simulink library "halin"  (R2021b)
settings: Solver=VariableStepAuto  StartTime=0.0  StopTime=10.0  RelTol=1e-3
undefined symbols (not defined in the file): KHAL_CAN1ABM1E2E_flg, KHAL_CAN1EPB1E2E_flg, KHAL_CAN1EPS1E2E_flg, KHAL_CAN1ESC1E2E_flg, KHAL_CAN1ESC5E2E_flg, KHAL_CAN3BMS1E2E_flg, KHAL_CAN3BMS6E2E_flg, KHAL_CAN3CCU1E2E_flg, KHAL_CAN3CCU2E2E_flg, KHAL_CAN3MCUNF1E2E_flg, KHAL_CAN3MCUNR1E2E_flg, KHAL_CAN3Shifter1E2E_flg, KHAL_CAN3Shifter2E2E_flg, KHAL_CAN6FCM2E2E_flg, KHAL_CAN6FCM4E2E_flg, TRUE
libraries: simulink x645, FVT_lib x212, hcu_lib x59
(part 20 of 23)

== system halin/HAL_IN/CAN3/CCU2/DCDCReady4Pre ==
  DCDCReady4Pre : Inport
  UnitConverter : DataTypeConversion  OutDataTypeStr=uint8
  VHAL_DCDCReady4Pre_flg : Outport
  wires:
  UnitConverter/1 -> VHAL_DCDCReady4Pre_flg/1
  DCDCReady4Pre/1 -> UnitConverter/1

== system halin/HAL_IN/CAN3/CCU2/DCDCTemp ==
  DCDCTemp : Inport
  UnitConverter : DataTypeConversion  OutDataTypeStr=uint8
  convert_in : FVT_lib/hal/convert_in  gain=0.75  offset=-48
  VHAL_DCDCTemp_C : Outport
  wires:
  convert_in/1 -> VHAL_DCDCTemp_C/1
  UnitConverter/1 -> convert_in/1
  DCDCTemp/1 -> UnitConverter/1

== system halin/HAL_IN/CAN3/CCU2/OBCACCurLim ==
  OBC_AC_Cur_Lim : Inport
  UnitConverter : DataTypeConversion  OutDataTypeStr=uint8
  VHAL_OBCACCurLim_enum : Outport
  wires:
  UnitConverter/1 -> VHAL_OBCACCurLim_enum/1
  OBC_AC_Cur_Lim/1 -> UnitConverter/1

== system halin/HAL_IN/CAN3/CCU2/OBCACCurrInf ==
  OBCACCurrInf : Inport
  UnitConverter : DataTypeConversion  OutDataTypeStr=uint16
  convert_in : FVT_lib/hal/convert_in  gain=0.125  offset=-40
  VHAL_OBCACCurrInf_A : Outport
  wires:
  convert_in/1 -> VHAL_OBCACCurrInf_A/1
  UnitConverter/1 -> convert_in/1
  OBCACCurrInf/1 -> UnitConverter/1

== system halin/HAL_IN/CAN3/CCU2/OBCACVoltInf ==
  OBCACVoltInf : Inport
  UnitConverter : DataTypeConversion  OutDataTypeStr=uint16
  convert_in : FVT_lib/hal/convert_in  gain=0.1  offset=0
  VHAL_OBCACVoltInf_V : Outport
  wires:
  convert_in/1 -> VHAL_OBCACVoltInf_V/1
  UnitConverter/1 -> convert_in/1
  OBCACVoltInf/1 -> UnitConverter/1

== system halin/HAL_IN/CAN3/CCU2/OBCEnaSta ==
  OBCEnaSta : Inport
  UnitConverter : DataTypeConversion  OutDataTypeStr=uint8
  VHAL_OBCEnaSta_flg : Outport
  wires:
  UnitConverter/1 -> VHAL_OBCEnaSta_flg/1
  OBCEnaSta/1 -> UnitConverter/1

== system halin/HAL_IN/CAN3/CCU2/OBCFaultSta ==
  OBCFaultSta : Inport
  UnitConverter : DataTypeConversion  OutDataTypeStr=uint8
  VHAL_OBCFaultSta_enum : Outport
  wires:
  UnitConverter/1 -> VHAL_OBCFaultSta_enum/1
  OBCFaultSta/1 -> UnitConverter/1

== system halin/HAL_IN/CAN3/CCU2/OBCPluginSta ==
  OBCPluginSta : Inport
  UnitConverter : DataTypeConversion  OutDataTypeStr=uint8
  VHAL_OBCPluginSta_flg : Outport
  wires:
  UnitConverter/1 -> VHAL_OBCPluginSta_flg/1
  OBCPluginSta/1 -> UnitConverter/1

== system halin/HAL_IN/CAN3/CCU2/OBCReady4Pre ==
  OBCReady4Pre : Inport
  UnitConverter : DataTypeConversion  OutDataTypeStr=uint8
  VHAL_OBCReady4Pre_flg : Outport
  wires:
  UnitConverter/1 -> VHAL_OBCReady4Pre_flg/1
  OBCReady4Pre/1 -> UnitConverter/1

== system halin/HAL_IN/CAN3/CCU2/OBCTemp ==
  OBCTemp : Inport
  UnitConverter : DataTypeConversion  OutDataTypeStr=uint16
  convert_in : FVT_lib/hal/convert_in  gain=0.3  offset=-48
  VHAL_OBCTemp_C : Outport
  wires:
  convert_in/1 -> VHAL_OBCTemp_C/1
  UnitConverter/1 -> convert_in/1
  OBCTemp/1 -> UnitConverter/1

== system halin/HAL_IN/CAN3/CCU2/OBCV2LSta ==
  OBCV2LSta : Inport
  UnitConverter : DataTypeConversion  OutDataTypeStr=uint8
  VHAL_OBCV2LSta_enum : Outport
  wires:
  UnitConverter/1 -> VHAL_OBCV2LSta_enum/1
  OBCV2LSta/1 -> UnitConverter/1

== system halin/HAL_IN/CAN3/CCU2/RCCCU2 ==
  RC_CCU2 : Inport
  UnitConverter : DataTypeConversion  OutDataTypeStr=uint8
  VHAL_RCCCU2_enum : Outport
  wires:
  UnitConverter/1 -> VHAL_RCCCU2_enum/1
  RC_CCU2/1 -> UnitConverter/1

== system halin/HAL_IN/CAN3/EBM1/EBMErrSta ==
  EBMErrSta : Inport
  UnitConverter : DataTypeConversion  OutDataTypeStr=uint8
  VHAL_EBMErrSta_enum : Outport
  wires:
  UnitConverter/1 -> VHAL_EBMErrSta_enum/1
  EBMErrSta/1 -> UnitConverter/1

== system halin/HAL_IN/CAN3/EBM1/EBMRLampSta ==
  EBMRLampSta : Inport
  UnitConverter : DataTypeConversion  OutDataTypeStr=uint8
  VHAL_EBMRLampSta_enum : Outport
  wires:
  UnitConverter/1 -> VHAL_EBMRLampSta_enum/1
  EBMRLampSta/1 -> UnitConverter/1

== system halin/HAL_IN/CAN3/MCU_B_F1/FrActvDmpDisabSta ==
  Fr_ActvDmpDisabSta : Inport
  UnitConverter : DataTypeConversion  OutDataTypeStr=uint8
  VHAL_FrActvDmpDisabSta_flg : Outport
  wires:
  UnitConverter/1 -> VHAL_FrActvDmpDisabSta_flg/1
  Fr_ActvDmpDisabSta/1 -> UnitConverter/1

== system halin/HAL_IN/CAN3/MCU_B_F1/FrEDUDrtSta ==
  Fr_EDUDrtSta : Inport
  UnitConverter : DataTypeConversion  OutDataTypeStr=uint8
  VHAL_FrEDUDrtSta_flg : Outport
  wires:
  UnitConverter/1 -> VHAL_FrEDUDrtSta_flg/1
  Fr_EDUDrtSta/1 -> UnitConverter/1

== system halin/HAL_IN/CAN3/MCU_B_F1/FrEDUOpratingSta ==
  Fr_EDUOpratingSta : Inport
  UnitConverter : DataTypeConversion  OutDataTypeStr=uint8
  VHAL_FrEDUOpratingSta_flg : Outport
  wires:
  UnitConverter/1 -> VHAL_FrEDUOpratingSta_flg/1
  Fr_EDUOpratingSta/1 -> UnitConverter/1

== system halin/HAL_IN/CAN3/MCU_B_F1/FrEDURealTMTq ==
  Fr_EDURealTMTq : Inport
  UnitConverter : DataTypeConversion  OutDataTypeStr=uint16
  convert_in : FVT_lib/hal/convert_in  gain=0.1  offset=-1022
  VHAL_FrEDURealTMTq_Nm : Outport
  wires:
  convert_in/1 -> VHAL_FrEDURealTMTq_Nm/1
  UnitConverter/1 -> convert_in/1
  Fr_EDURealTMTq/1 -> UnitConverter/1

== system halin/HAL_IN/CAN3/MCU_B_F1/FrEDURotateDirction ==
  Fr_EDURotateDirction : Inport
  UnitConverter : DataTypeConversion  OutDataTypeStr=uint8
  VHAL_FrEDURotateDirction_enum : Outport
  wires:
  UnitConverter/1 -> VHAL_FrEDURotateDirction_enum/1
  Fr_EDURotateDirction/1 -> UnitConverter/1

== system halin/HAL_IN/CAN3/MCU_B_F1/FrEDUTqReqFbk ==
  Fr_EDUTqReqFbk : Inport
  UnitConverter : DataTypeConversion  OutDataTypeStr=uint16
  convert_in : FVT_lib/hal/convert_in  gain=1  offset=-1022
  VHAL_FrEDUTqReqFbk_Nm : Outport
  wires:
  convert_in/1 -> VHAL_FrEDUTqReqFbk_Nm/1
  UnitConverter/1 -> convert_in/1
  Fr_EDUTqReqFbk/1 -> UnitConverter/1

== system halin/HAL_IN/CAN3/MCU_B_F1/FrMCUBAT ==
  Fr_MCUBAT : Inport
  UnitConverter : DataTypeConversion  OutDataTypeStr=uint8
  convert_in : FVT_lib/hal/convert_in  gain=0.1  offset=0
  VHAL_FrMCUBAT_V : Outport
  wires:
  convert_in/1 -> VHAL_FrMCUBAT_V/1
  UnitConverter/1 -> convert_in/1
  Fr_MCUBAT/1 -> UnitConverter/1

== system halin/HAL_IN/CAN3/MCU_B_F1/FrMCUDCBusCurr ==
  Fr_MCUDCBusCurr : Inport
  UnitConverter : DataTypeConversion  OutDataTypeStr=uint16
  convert_in : FVT_lib/hal/convert_in  gain=0.1  offset=-1500
  VHAL_FrMCUDCBusCurr_A : Outport
  wires:
  convert_in/1 -> VHAL_FrMCUDCBusCurr_A/1
  UnitConverter/1 -> convert_in/1
  Fr_MCUDCBusCurr/1 -> UnitConverter/1

== system halin/HAL_IN/CAN3/MCU_B_F1/FrMCUDCBusVolt ==
  Fr_MCUDCBusVolt : Inport
  UnitConverter : DataTypeConversion  OutDataTypeStr=uint16
  convert_in : FVT_lib/hal/convert_in  gain=0.1  offset=0
  VHAL_FrMCUDCBusVolt_V : Outport
  wires:
  convert_in/1 -> VHAL_FrMCUDCBusVolt_V/1
  UnitConverter/1 -> convert_in/1
  Fr_MCUDCBusVolt/1 -> UnitConverter/1

== system halin/HAL_IN/CAN3/MCU_B_F1/FrMCUDischrgSta ==
  Fr_MCUDischrgSta : Inport
  UnitConverter : DataTypeConversion  OutDataTypeStr=uint8
  VHAL_FrMCUDischrgSta_flg : Outport
  wires:
  UnitConverter/1 -> VHAL_FrMCUDischrgSta_flg/1
  Fr_MCUDischrgSta/1 -> UnitConverter/1

== system halin/HAL_IN/CAN3/MCU_B_F1/FrMCUEnaSta ==
  Fr_MCUEnaSta : Inport
  UnitConverter : DataTypeConversion  OutDataTypeStr=uint8
  VHAL_FrMCUEnaSta_flg : Outport
  wires:
  UnitConverter/1 -> VHAL_FrMCUEnaSta_flg/1
  Fr_MCUEnaSta/1 -> UnitConverter/1

== system halin/HAL_IN/CAN3/MCU_B_F1/FrMCUErr ==
  Fr_MCUErr : Inport
  UnitConverter : DataTypeConversion  OutDataTypeStr=uint8
  VHAL_FrMCUErr_enum : Outport
  wires:
  UnitConverter/1 -> VHAL_FrMCUErr_enum/1
  Fr_MCUErr/1 -> UnitConverter/1

== system halin/HAL_IN/CAN3/MCU_B_F1/FrMCUIGNsta ==
  Fr_MCUIGN_sta : Inport
  UnitConverter : DataTypeConversion  OutDataTypeStr=uint8
  VHAL_FrMCUIGNsta_flg : Outport
  wires:
  UnitConverter/1 -> VHAL_FrMCUIGNsta_flg/1
  Fr_MCUIGN_sta/1 -> UnitConverter/1

== system halin/HAL_IN/CAN3/MCU_B_F1/FrMCUReady ==
  Fr_MCUReady : Inport
  UnitConverter : DataTypeConversion  OutDataTypeStr=uint8
  VHAL_FrMCUReady_flg : Outport
  wires:
  UnitConverter/1 -> VHAL_FrMCUReady_flg/1
  Fr_MCUReady/1 -> UnitConverter/1

== system halin/HAL_IN/CAN3/MCU_B_F1/FrMCUReady4Pre ==
  Fr_MCUReady4Pre : Inport
  UnitConverter : DataTypeConversion  OutDataTypeStr=uint8
  VHAL_FrMCUReady4Pre_flg : Outport
  wires:
  UnitConverter/1 -> VHAL_FrMCUReady4Pre_flg/1
  Fr_MCUReady4Pre/1 -> UnitConverter/1

== system halin/HAL_IN/CAN3/MCU_B_F1/FrMCUSysSta ==
  Fr_MCUSysSta : Inport
  UnitConverter : DataTypeConversion  OutDataTypeStr=uint8
  VHAL_FrMCUSysSta_enum : Outport
  wires:
  UnitConverter/1 -> VHAL_FrMCUSysSta_enum/1
  Fr_MCUSysSta/1 -> UnitConverter/1

== system halin/HAL_IN/CAN3/MCU_B_F1/FrMCUTemp ==
  Fr_MCUTemp : Inport
  UnitConverter : DataTypeConversion  OutDataTypeStr=uint16
  convert_in : FVT_lib/hal/convert_in  gain=1  offset=-40
  VHAL_FrMCUTemp_C : Outport
  wires:
  convert_in/1 -> VHAL_FrMCUTemp_C/1
  UnitConverter/1 -> convert_in/1
  Fr_MCUTemp/1 -> UnitConverter/1

== system halin/HAL_IN/CAN3/MCU_B_F1/FrMotorAvailTq ==
  Fr_MotorAvailTq : Inport
  UnitConverter : DataTypeConversion  OutDataTypeStr=uint16
  VHAL_FrMotorAvailTq_Nm : Outport
  wires:
  UnitConverter/1 -> VHAL_FrMotorAvailTq_Nm/1
  Fr_MotorAvailTq/1 -> UnitConverter/1

== system halin/HAL_IN/CAN3/MCU_B_F1/FrRegenAvailTq ==
  Fr_RegenAvailTq : Inport
  UnitConverter : DataTypeConversion  OutDataTypeStr=uint16
  convert_in : FVT_lib/hal/convert_in  gain=1  offset=-1022
  VHAL_FrRegenAvailTq_Nm : Outport
  wires:
  convert_in/1 -> VHAL_FrRegenAvailTq_Nm/1
  UnitConverter/1 -> convert_in/1
  Fr_RegenAvailTq/1 -> UnitConverter/1

== system halin/HAL_IN/CAN3/MCU_B_F1/FrTMSpd ==
  Fr_TMSpd : Inport
  UnitConverter : DataTypeConversion  OutDataTypeStr=uint16
  convert_in : FVT_lib/hal/convert_in  gain=1  offset=-18000
  VHAL_FrTMSpd_rpm : Outport
  wires:
  convert_in/1 -> VHAL_FrTMSpd_rpm/1
  UnitConverter/1 -> convert_in/1
  Fr_TMSpd/1 -> UnitConverter/1

== system halin/HAL_IN/CAN3/MCU_B_F1/FrTMTemp ==
  Fr_TMTemp : Inport
  UnitConverter : DataTypeConversion  OutDataTypeStr=uint16
  convert_in : FVT_lib/hal/convert_in  gain=1  offset=-40
  VHAL_FrTMTemp_C : Outport
  wires:
  convert_in/1 -> VHAL_FrTMTemp_C/1
  UnitConverter/1 -> convert_in/1
  Fr_TMTemp/1 -> UnitConverter/1

== system halin/HAL_IN/CAN3/MCU_B_F1/FrTMid ==
  Fr_TMid : Inport
  UnitConverter : DataTypeConversion  OutDataTypeStr=uint16
  convert_in : FVT_lib/hal/convert_in  gain=0.1  offset=-1500
  VHAL_FrTMid_A : Outport
  wires:
  convert_in/1 -> VHAL_FrTMid_A/1
  UnitConverter/1 -> convert_in/1
  Fr_TMid/1 -> UnitConverter/1

== system halin/HAL_IN/CAN3/MCU_B_F1/FrTMiq ==
  Fr_TMiq : Inport
  UnitConverter : DataTypeConversion  OutDataTypeStr=uint16
  convert_in : FVT_lib/hal/convert_in  gain=0.1  offset=-1500
  VHAL_FrTMiq_A : Outport
  wires:
  convert_in/1 -> VHAL_FrTMiq_A/1
  UnitConverter/1 -> convert_in/1
  Fr_TMiq/1 -> UnitConverter/1

== system halin/HAL_IN/CAN3/MCU_B_F1/MCUBFRealPwrKwSta ==
  MCU_B_F_RealPwrKw_Sta : Inport
  UnitConverter : DataTypeConversion  OutDataTypeStr=uint16
  convert_in : FVT_lib/hal/convert_in  gain=0.1  offset=-530
  VHAL_MCUBFRealPwrKwSta_kW : Outport
  wires:
  convert_in/1 -> VHAL_MCUBFRealPwrKwSta_kW/1
  UnitConverter/1 -> convert_in/1
  MCU_B_F_RealPwrKw_Sta/1 -> UnitConverter/1

== system halin/HAL_IN/CAN3/MCU_B_F1/MCUWarnF ==
  MCUWarn_F : Inport
  UnitConverter : DataTypeConversion  OutDataTypeStr=uint8
  VHAL_MCUWarnF_enum : Outport
  wires:
  UnitConverter/1 -> VHAL_MCUWarnF_enum/1
  MCUWarn_F/1 -> UnitConverter/1

== system halin/HAL_IN/CAN3/MCU_B_F2/FrCoolanttempReq ==
  Fr_CoolanttempReq : Inport
  UnitConverter : DataTypeConversion  OutDataTypeStr=uint16
  convert_in : FVT_lib/hal/convert_in  gain=1  offset=-40
  VHAL_FrCoolanttempReq_C : Outport
  wires:
  convert_in/1 -> VHAL_FrCoolanttempReq_C/1
  UnitConverter/1 -> convert_in/1
  Fr_CoolanttempReq/1 -> UnitConverter/1

== system halin/HAL_IN/CAN3/MCU_B_F2/FrFailcode1 ==
  Fr_Failcode1 : Inport
  UnitConverter : DataTypeConversion  OutDataTypeStr=uint8
  VHAL_FrFailcode1_enum : Outport
  wires:
  UnitConverter/1 -> VHAL_FrFailcode1_enum/1
  Fr_Failcode1/1 -> UnitConverter/1

== system halin/HAL_IN/CAN3/MCU_B_F2/FrFailcode2 ==
  Fr_Failcode2 : Inport
  UnitConverter : DataTypeConversion  OutDataTypeStr=uint8
  VHAL_FrFailcode2_enum : Outport
  wires:
  UnitConverter/1 -> VHAL_FrFailcode2_enum/1
  Fr_Failcode2/1 -> UnitConverter/1

== system halin/HAL_IN/CAN3/MCU_B_F2/FrFailcodehistory1 ==
  Fr_Failcodehistory1 : Inport
  UnitConverter : DataTypeConversion  OutDataTypeStr=uint8
  VHAL_FrFailcodehistory1_enum : Outport
  wires:
  UnitConverter/1 -> VHAL_FrFailcodehistory1_enum/1
  Fr_Failcodehistory1/1 -> UnitConverter/1

== system halin/HAL_IN/CAN3/MCU_B_F2/FrFailcodehistory2 ==
  Fr_Failcodehistory2 : Inport
  UnitConverter : DataTypeConversion  OutDataTypeStr=uint8
  VHAL_FrFailcodehistory2_enum : Outport
  wires:
  UnitConverter/1 -> VHAL_FrFailcodehistory2_enum/1
  Fr_Failcodehistory2/1 -> UnitConverter/1

== system halin/HAL_IN/CAN3/MCU_B_F2/FrLLCTemp ==
  Fr_LLCTemp : Inport
  UnitConverter : DataTypeConversion  OutDataTypeStr=uint16
  convert_in : FVT_lib/hal/convert_in  gain=1  offset=-40
  VHAL_FrLLCTemp_C : Outport
  wires:
  convert_in/1 -> VHAL_FrLLCTemp_C/1
  UnitConverter/1 -> convert_in/1
  Fr_LLCTemp/1 -> UnitConverter/1

== system halin/HAL_IN/CAN3/MCU_B_F2/FrLLCflowReq ==
  Fr_LLCflowReq : Inport
  UnitConverter : DataTypeConversion  OutDataTypeStr=uint8
  convert_in : FVT_lib/hal/convert_in  gain=0.25  offset=0
  VHAL_FrLLCflowReq_Lpmin : Outport
  wires:
  convert_in/1 -> VHAL_FrLLCflowReq_Lpmin/1
  UnitConverter/1 -> convert_in/1
  Fr_LLCflowReq/1 -> UnitConverter/1

== system halin/HAL_IN/CAN3/MCU_B_F2/FrMCUHWVer ==
  Fr_MCU_HW_Ver : Inport
  UnitConverter : DataTypeConversion  OutDataTypeStr=uint16
  VHAL_FrMCUHWVer_enum : Outport
  wires:
  UnitConverter/1 -> VHAL_FrMCUHWVer_enum/1
  Fr_MCU_HW_Ver/1 -> UnitConverter/1

== system halin/HAL_IN/CAN3/MCU_B_F2/FrMCUSWVer ==
  Fr_MCU_SW_Ver : Inport
  UnitConverter : DataTypeConversion  OutDataTypeStr=uint16
  VHAL_FrMCUSWVer_enum : Outport
  wires:
  UnitConverter/1 -> VHAL_FrMCUSWVer_enum/1
  Fr_MCU_SW_Ver/1 -> UnitConverter/1

== system halin/HAL_IN/CAN3/MCU_B_F2/FrMCUTempWarn ==
  Fr_MCUTempWarn : Inport
  UnitConverter : DataTypeConversion  OutDataTypeStr=uint8
  VHAL_FrMCUTempWarn_enum : Outport
  wires:
  UnitConverter/1 -> VHAL_FrMCUTempWarn_enum/1
  Fr_MCUTempWarn/1 -> UnitConverter/1

== system halin/HAL_IN/CAN3/MCU_B_F2/FrTMTempWarn ==
  Fr_TMTempWarn : Inport
  UnitConverter : DataTypeConversion  OutDataTypeStr=uint8
  VHAL_FrTMTempWarn_enum : Outport
  wires:
  UnitConverter/1 -> VHAL_FrTMTempWarn_enum/1
  Fr_TMTempWarn/1 -> UnitConverter/1

== system halin/HAL_IN/CAN3/MCU_B_F2/MCUBFLLCTempWarnSta ==
  MCU_B_F_LLCTempWarn_Sta : Inport
  UnitConverter : DataTypeConversion  OutDataTypeStr=uint8
  VHAL_MCUBFLLCTempWarnSta_enum : Outport
  wires:
  UnitConverter/1 -> VHAL_MCUBFLLCTempWarnSta_enum/1
  MCU_B_F_LLCTempWarn_Sta/1 -> UnitConverter/1

== system halin/HAL_IN/CAN3/MCU_B_R1/MCUBRRealPwrKwSta ==
  MCU_B_R_RealPwrKw_Sta : Inport
  UnitConverter : DataTypeConversion  OutDataTypeStr=uint16
  convert_in : FVT_lib/hal/convert_in  gain=0.1  offset=-530
  VHAL_MCUBRRealPwrKwSta_kW : Outport
  wires:
  convert_in/1 -> VHAL_MCUBRRealPwrKwSta_kW/1
  UnitConverter/1 -> convert_in/1
  MCU_B_R_RealPwrKw_Sta/1 -> UnitConverter/1

== system halin/HAL_IN/CAN3/MCU_B_R1/MCUWarnR ==
  MCUWarn_R : Inport
  UnitConverter : DataTypeConversion  OutDataTypeStr=uint8
  VHAL_MCUWarnR_enum : Outport
  wires:
  UnitConverter/1 -> VHAL_MCUWarnR_enum/1
  MCUWarn_R/1 -> UnitConverter/1

== system halin/HAL_IN/CAN3/MCU_B_R1/RrActvDmpDisabSta ==
  Rr_ActvDmpDisabSta : Inport
  UnitConverter : DataTypeConversion  OutDataTypeStr=uint8
  VHAL_RrActvDmpDisabSta_flg : Outport
  wires:
  UnitConverter/1 -> VHAL_RrActvDmpDisabSta_flg/1
  Rr_ActvDmpDisabSta/1 -> UnitConverter/1

== system halin/HAL_IN/CAN3/MCU_B_R1/RrEDUDrtSta ==
  Rr_EDUDrtSta : Inport
  UnitConverter : DataTypeConversion  OutDataTypeStr=uint8
  VHAL_RrEDUDrtSta_flg : Outport
  wires:
  UnitConverter/1 -> VHAL_RrEDUDrtSta_flg/1
  Rr_EDUDrtSta/1 -> UnitConverter/1

== system halin/HAL_IN/CAN3/MCU_B_R1/RrEDUOpratingSta ==
  Rr_EDUOpratingSta : Inport
  UnitConverter : DataTypeConversion  OutDataTypeStr=uint8
  VHAL_RrEDUOpratingSta_flg : Outport
  wires:
  UnitConverter/1 -> VHAL_RrEDUOpratingSta_flg/1
  Rr_EDUOpratingSta/1 -> UnitConverter/1

== system halin/HAL_IN/CAN3/MCU_B_R1/RrEDURealTMTq ==
  Rr_EDURealTMTq : Inport
  UnitConverter : DataTypeConversion  OutDataTypeStr=uint16
  convert_in : FVT_lib/hal/convert_in  gain=0.1  offset=-1022
  VHAL_RrEDURealTMTq_Nm : Outport
  wires:
  convert_in/1 -> VHAL_RrEDURealTMTq_Nm/1
  UnitConverter/1 -> convert_in/1
  Rr_EDURealTMTq/1 -> UnitConverter/1

== system halin/HAL_IN/CAN3/MCU_B_R1/RrEDURotateDirction ==
  Rr_EDURotateDirction : Inport
  UnitConverter : DataTypeConversion  OutDataTypeStr=uint8
  VHAL_RrEDURotateDirction_enum : Outport
  wires:
  UnitConverter/1 -> VHAL_RrEDURotateDirction_enum/1
  Rr_EDURotateDirction/1 -> UnitConverter/1

== system halin/HAL_IN/CAN3/MCU_B_R1/RrEDUTqReqFbk ==
  Rr_EDUTqReqFbk : Inport
  UnitConverter : DataTypeConversion  OutDataTypeStr=uint16
  convert_in : FVT_lib/hal/convert_in  gain=1  offset=-1022
  VHAL_RrEDUTqReqFbk_Nm : Outport
  wires:
  convert_in/1 -> VHAL_RrEDUTqReqFbk_Nm/1
  UnitConverter/1 -> convert_in/1
  Rr_EDUTqReqFbk/1 -> UnitConverter/1

== system halin/HAL_IN/CAN3/MCU_B_R1/RrMCUBAT ==
  Rr_MCUBAT : Inport
  UnitConverter : DataTypeConversion  OutDataTypeStr=uint8
  convert_in : FVT_lib/hal/convert_in  gain=0.1  offset=0
  VHAL_RrMCUBAT_V : Outport
  wires:
  convert_in/1 -> VHAL_RrMCUBAT_V/1
  UnitConverter/1 -> convert_in/1
  Rr_MCUBAT/1 -> UnitConverter/1

== system halin/HAL_IN/CAN3/MCU_B_R1/RrMCUDCBusCurr ==
  Rr_MCUDCBusCurr : Inport
  UnitConverter : DataTypeConversion  OutDataTypeStr=uint16
  convert_in : FVT_lib/hal/convert_in  gain=0.1  offset=-1500
  VHAL_RrMCUDCBusCurr_A : Outport
  wires:
  convert_in/1 -> VHAL_RrMCUDCBusCurr_A/1
  UnitConverter/1 -> convert_in/1
  Rr_MCUDCBusCurr/1 -> UnitConverter/1

== system halin/HAL_IN/CAN3/MCU_B_R1/RrMCUDCBusVolt ==
  Rr_MCUDCBusVolt : Inport
  UnitConverter : DataTypeConversion  OutDataTypeStr=uint16
  convert_in : FVT_lib/hal/convert_in  gain=0.1  offset=0
  VHAL_RrMCUDCBusVolt_V : Outport
  wires:
  convert_in/1 -> VHAL_RrMCUDCBusVolt_V/1
  UnitConverter/1 -> convert_in/1
  Rr_MCUDCBusVolt/1 -> UnitConverter/1

== system halin/HAL_IN/CAN3/MCU_B_R1/RrMCUDischrgSta ==
  Rr_MCUDischrgSta : Inport
  UnitConverter : DataTypeConversion  OutDataTypeStr=uint8
  VHAL_RrMCUDischrgSta_flg : Outport
  wires:
  UnitConverter/1 -> VHAL_RrMCUDischrgSta_flg/1
  Rr_MCUDischrgSta/1 -> UnitConverter/1

== system halin/HAL_IN/CAN3/MCU_B_R1/RrMCUEnaSta ==
  Rr_MCUEnaSta : Inport
  UnitConverter : DataTypeConversion  OutDataTypeStr=uint8
  VHAL_RrMCUEnaSta_flg : Outport
  wires:
  UnitConverter/1 -> VHAL_RrMCUEnaSta_flg/1
  Rr_MCUEnaSta/1 -> UnitConverter/1

== system halin/HAL_IN/CAN3/MCU_B_R1/RrMCUErr ==
  Rr_MCUErr : Inport
  UnitConverter : DataTypeConversion  OutDataTypeStr=uint8
  VHAL_RrMCUErr_enum : Outport
  wires:
  UnitConverter/1 -> VHAL_RrMCUErr_enum/1
  Rr_MCUErr/1 -> UnitConverter/1

== system halin/HAL_IN/CAN3/MCU_B_R1/RrMCUIGNsta ==
  Rr_MCUIGN_sta : Inport
  UnitConverter : DataTypeConversion  OutDataTypeStr=uint8
  VHAL_RrMCUIGNsta_flg : Outport
  wires:
  UnitConverter/1 -> VHAL_RrMCUIGNsta_flg/1
  Rr_MCUIGN_sta/1 -> UnitConverter/1

== system halin/HAL_IN/CAN3/MCU_B_R1/RrMCUReady ==
  Rr_MCUReady : Inport
  UnitConverter : DataTypeConversion  OutDataTypeStr=uint8
  VHAL_RrMCUReady_flg : Outport
  wires:
  UnitConverter/1 -> VHAL_RrMCUReady_flg/1
  Rr_MCUReady/1 -> UnitConverter/1

== system halin/HAL_IN/CAN3/MCU_B_R1/RrMCUReady4Pre ==
  Rr_MCUReady4Pre : Inport
  UnitConverter : DataTypeConversion  OutDataTypeStr=uint8
  VHAL_RrMCUReady4Pre_flg : Outport
  wires:
  UnitConverter/1 -> VHAL_RrMCUReady4Pre_flg/1
  Rr_MCUReady4Pre/1 -> UnitConverter/1

== system halin/HAL_IN/CAN3/MCU_B_R1/RrMCUSysSta ==
  Rr_MCUSysSta : Inport
  UnitConverter : DataTypeConversion  OutDataTypeStr=uint8
  VHAL_RrMCUSysSta_enum : Outport
  wires:
  UnitConverter/1 -> VHAL_RrMCUSysSta_enum/1
  Rr_MCUSysSta/1 -> UnitConverter/1

== system halin/HAL_IN/CAN3/MCU_B_R1/RrMCUTemp ==
  Rr_MCUTemp : Inport
  UnitConverter : DataTypeConversion  OutDataTypeStr=uint16
  convert_in : FVT_lib/hal/convert_in  gain=1  offset=-40
  VHAL_RrMCUTemp_C : Outport
  wires:
  convert_in/1 -> VHAL_RrMCUTemp_C/1
  UnitConverter/1 -> convert_in/1
  Rr_MCUTemp/1 -> UnitConverter/1

== system halin/HAL_IN/CAN3/MCU_B_R1/RrMotorAvailTq ==
  Rr_MotorAvailTq : Inport
  UnitConverter : DataTypeConversion  OutDataTypeStr=uint16
  VHAL_RrMotorAvailTq_Nm : Outport
  wires:
  UnitConverter/1 -> VHAL_RrMotorAvailTq_Nm/1
  Rr_MotorAvailTq/1 -> UnitConverter/1

== system halin/HAL_IN/CAN3/MCU_B_R1/RrRegenAvailTq ==
  Rr_RegenAvailTq : Inport
  UnitConverter : DataTypeConversion  OutDataTypeStr=uint16
  convert_in : FVT_lib/hal/convert_in  gain=1  offset=-1022
  VHAL_RrRegenAvailTq_Nm : Outport
  wires:
  convert_in/1 -> VHAL_RrRegenAvailTq_Nm/1
  UnitConverter/1 -> convert_in/1
  Rr_RegenAvailTq/1 -> UnitConverter/1

== system halin/HAL_IN/CAN3/MCU_B_R1/RrTMSpd ==
  Rr_TMSpd : Inport
  UnitConverter : DataTypeConversion  OutDataTypeStr=uint16
  convert_in : FVT_lib/hal/convert_in  gain=1  offset=-18000
  VHAL_RrTMSpd_rpm : Outport
  wires:
  convert_in/1 -> VHAL_RrTMSpd_rpm/1
  UnitConverter/1 -> convert_in/1
  Rr_TMSpd/1 -> UnitConverter/1

== system halin/HAL_IN/CAN3/MCU_B_R1/RrTMTemp ==
  Rr_TMTemp : Inport
  UnitConverter : DataTypeConversion  OutDataTypeStr=uint16
  convert_in : FVT_lib/hal/convert_in  gain=1  offset=-40
  VHAL_RrTMTemp_C : Outport
  wires:
  convert_in/1 -> VHAL_RrTMTemp_C/1
  UnitConverter/1 -> convert_in/1
  Rr_TMTemp/1 -> UnitConverter/1

== system halin/HAL_IN/CAN3/MCU_B_R1/RrTMid ==
  Rr_TMid : Inport
  UnitConverter : DataTypeConversion  OutDataTypeStr=uint16
  convert_in : FVT_lib/hal/convert_in  gain=0.1  offset=-1500
  VHAL_RrTMid_A : Outport
  wires:
  convert_in/1 -> VHAL_RrTMid_A/1
  UnitConverter/1 -> convert_in/1
  Rr_TMid/1 -> UnitConverter/1

== system halin/HAL_IN/CAN3/MCU_B_R1/RrTMiq ==
  Rr_TMiq : Inport
  UnitConverter : DataTypeConversion  OutDataTypeStr=uint16
  convert_in : FVT_lib/hal/convert_in  gain=0.1  offset=-1500
  VHAL_RrTMiq_A : Outport
  wires:
  convert_in/1 -> VHAL_RrTMiq_A/1
  UnitConverter/1 -> convert_in/1
  Rr_TMiq/1 -> UnitConverter/1

== system halin/HAL_IN/CAN3/MCU_B_R2/MCUBRLLCTempWarnSta ==
  MCU_B_R_LLCTempWarn_Sta : Inport
  UnitConverter : DataTypeConversion  OutDataTypeStr=uint8
  VHAL_MCUBRLLCTempWarnSta_enum : Outport
  wires:
  UnitConverter/1 -> VHAL_MCUBRLLCTempWarnSta_enum/1
  MCU_B_R_LLCTempWarn_Sta/1 -> UnitConverter/1

== system halin/HAL_IN/CAN3/MCU_B_R2/RrCoolanttempReq ==
  Rr_CoolanttempReq : Inport
  UnitConverter : DataTypeConversion  OutDataTypeStr=uint16
  convert_in : FVT_lib/hal/convert_in  gain=1  offset=-40
  VHAL_RrCoolanttempReq_cnt : Outport
  wires:
  convert_in/1 -> VHAL_RrCoolanttempReq_cnt/1
  UnitConverter/1 -> convert_in/1
  Rr_CoolanttempReq/1 -> UnitConverter/1

== system halin/HAL_IN/CAN3/MCU_B_R2/RrFailcode1 ==
  Rr_Failcode1 : Inport
  UnitConverter : DataTypeConversion  OutDataTypeStr=uint8
  VHAL_RrFailcode1_enum : Outport
  wires:
  UnitConverter/1 -> VHAL_RrFailcode1_enum/1
  Rr_Failcode1/1 -> UnitConverter/1

== system halin/HAL_IN/CAN3/MCU_B_R2/RrFailcode2 ==
  Rr_Failcode2 : Inport
  UnitConverter : DataTypeConversion  OutDataTypeStr=uint8
  VHAL_RrFailcode2_enum : Outport
  wires:
  UnitConverter/1 -> VHAL_RrFailcode2_enum/1
  Rr_Failcode2/1 -> UnitConverter/1

== system halin/HAL_IN/CAN3/MCU_B_R2/RrFailcodehistory1 ==
  Rr_Failcodehistory1 : Inport
  UnitConverter : DataTypeConversion  OutDataTypeStr=uint8
  VHAL_RrFailcodehistory1_enum : Outport
  wires:
  UnitConverter/1 -> VHAL_RrFailcodehistory1_enum/1
  Rr_Failcodehistory1/1 -> UnitConverter/1

== system halin/HAL_IN/CAN3/MCU_B_R2/RrFailcodehistory2 ==
  Rr_Failcodehistory2 : Inport
  UnitConverter : DataTypeConversion  OutDataTypeStr=uint8
  VHAL_RrFailcodehistory2_enum : Outport
  wires:
  UnitConverter/1 -> VHAL_RrFailcodehistory2_enum/1
  Rr_Failcodehistory2/1 -> UnitConverter/1

== system halin/HAL_IN/CAN3/MCU_B_R2/RrLLCTemp ==
  Rr_LLCTemp : Inport
  UnitConverter : DataTypeConversion  OutDataTypeStr=uint16
  convert_in : FVT_lib/hal/convert_in  gain=1  offset=-40
  VHAL_RrLLCTemp_C : Outport
  wires:
  convert_in/1 -> VHAL_RrLLCTemp_C/1
  UnitConverter/1 -> convert_in/1
  Rr_LLCTemp/1 -> UnitConverter/1

== system halin/HAL_IN/CAN3/MCU_B_R2/RrLLCflowReq ==
  Rr_LLCflowReq : Inport
  UnitConverter : DataTypeConversion  OutDataTypeStr=uint8
  convert_in : FVT_lib/hal/convert_in  gain=0.25  offset=0
  VHAL_RrLLCflowReq_Lpmin : Outport
  wires:
  convert_in/1 -> VHAL_RrLLCflowReq_Lpmin/1
  UnitConverter/1 -> convert_in/1
  Rr_LLCflowReq/1 -> UnitConverter/1

== system halin/HAL_IN/CAN3/MCU_B_R2/RrMCU3HWVer ==
  Rr_MCU3_HW_Ver : Inport
  UnitConverter : DataTypeConversion  OutDataTypeStr=uint16
  VHAL_RrMCU3HWVer_enum : Outport
  wires:
  UnitConverter/1 -> VHAL_RrMCU3HWVer_enum/1
  Rr_MCU3_HW_Ver/1 -> UnitConverter/1

== system halin/HAL_IN/CAN3/MCU_B_R2/RrMCU3SWVer ==
  Rr_MCU3_SW_Ver : Inport
  UnitConverter : DataTypeConversion  OutDataTypeStr=uint16
  VHAL_RrMCU3SWVer_enum : Outport
  wires:
  UnitConverter/1 -> VHAL_RrMCU3SWVer_enum/1
  Rr_MCU3_SW_Ver/1 -> UnitConverter/1

== system halin/HAL_IN/CAN3/MCU_B_R2/RrMCUTempWarn ==
  Rr_MCUTempWarn : Inport
  UnitConverter : DataTypeConversion  OutDataTypeStr=uint8
  VHAL_RrMCUTempWarn_enum : Outport
  wires:
  UnitConverter/1 -> VHAL_RrMCUTempWarn_enum/1
  Rr_MCUTempWarn/1 -> UnitConverter/1

== system halin/HAL_IN/CAN3/MCU_B_R2/RrTMTempWarn ==
  Rr_TMTempWarn : Inport
  UnitConverter : DataTypeConversion  OutDataTypeStr=uint8
  VHAL_RrTMTempWarn_enum : Outport
  wires:
  UnitConverter/1 -> VHAL_RrTMTempWarn_enum/1
  Rr_TMTempWarn/1 -> UnitConverter/1

== system halin/HAL_IN/CAN3/MCU_N_F1/FrActvDmpDisabStaNidec ==
  Fr_ActvDmpDisabSta_Nidec : Inport
  UnitConverter : DataTypeConversion  OutDataTypeStr=uint8
  VHAL_FrActvDmpDisabStaNidec_flg : Outport
  wires:
  UnitConverter/1 -> VHAL_FrActvDmpDisabStaNidec_flg/1
  Fr_ActvDmpDisabSta_Nidec/1 -> UnitConverter/1

== system halin/HAL_IN/CAN3/MCU_N_F1/FrEDUDrtStaNidec ==
  Fr_EDUDrtSta_Nidec : Inport
  UnitConverter : DataTypeConversion  OutDataTypeStr=uint8
  VHAL_FrEDUDrtStaNidec_flg : Outport
  wires:
  UnitConverter/1 -> VHAL_FrEDUDrtStaNidec_flg/1
  Fr_EDUDrtSta_Nidec/1 -> UnitConverter/1

== system halin/HAL_IN/CAN3/MCU_N_F1/FrEDUOpratingStaNidec ==
  Fr_EDUOpratingSta_Nidec : Inport
  UnitConverter : DataTypeConversion  OutDataTypeStr=uint8
  VHAL_FrEDUOpratingStaNidec_flg : Outport
  wires:
  UnitConverter/1 -> VHAL_FrEDUOpratingStaNidec_flg/1
  Fr_EDUOpratingSta_Nidec/1 -> UnitConverter/1

== system halin/HAL_IN/CAN3/MCU_N_F1/FrEDURealTMTqNidec ==
  Fr_EDURealTMTq_Nidec : Inport
  UnitConverter : DataTypeConversion  OutDataTypeStr=uint16
  convert_in : FVT_lib/hal/convert_in  gain=1  offset=-1022
  VHAL_FrEDURealTMTqNidec_Nm : Outport
  wires:
  convert_in/1 -> VHAL_FrEDURealTMTqNidec_Nm/1
  UnitConverter/1 -> convert_in/1
  Fr_EDURealTMTq_Nidec/1 -> UnitConverter/1

== system halin/HAL_IN/CAN3/MCU_N_F1/FrEDURotateDirctionNidec ==
  Fr_EDURotateDirction_Nidec : Inport
  UnitConverter : DataTypeConversion  OutDataTypeStr=uint8
  VHAL_FrEDURotateDirctionNidec_enum : Outport
  wires:
  UnitConverter/1 -> VHAL_FrEDURotateDirctionNidec_enum/1
  Fr_EDURotateDirction_Nidec/1 -> UnitConverter/1

== system halin/HAL_IN/CAN3/MCU_N_F1/FrEDUTqReqFbkNidec ==
  Fr_EDUTqReqFbk_Nidec : Inport
  UnitConverter : DataTypeConversion  OutDataTypeStr=uint16
  convert_in : FVT_lib/hal/convert_in  gain=1  offset=-1022
  VHAL_FrEDUTqReqFbkNidec_Nm : Outport
  wires:
  convert_in/1 -> VHAL_FrEDUTqReqFbkNidec_Nm/1
  UnitConverter/1 -> convert_in/1
  Fr_EDUTqReqFbk_Nidec/1 -> UnitConverter/1

== system halin/HAL_IN/CAN3/MCU_N_F1/FrMCU1ChksumNidec ==
  Fr_MCU1Chksum_Nidec : Inport
  UnitConverter : DataTypeConversion  OutDataTypeStr=uint8
  VHAL_FrMCU1ChksumNidec_enum : Outport
  wires:
  UnitConverter/1 -> VHAL_FrMCU1ChksumNidec_enum/1
  Fr_MCU1Chksum_Nidec/1 -> UnitConverter/1

== system halin/HAL_IN/CAN3/MCU_N_F1/FrMCU1RolCntNidec ==
  Fr_MCU1RolCnt_Nidec : Inport
  UnitConverter : DataTypeConversion  OutDataTypeStr=uint8
  VHAL_FrMCU1RolCntNidec_enum : Outport
  wires:
  UnitConverter/1 -> VHAL_FrMCU1RolCntNidec_enum/1
  Fr_MCU1RolCnt_Nidec/1 -> UnitConverter/1

== system halin/HAL_IN/CAN3/MCU_N_F1/FrMCUBATNidec ==
  Fr_MCUBAT_Nidec : Inport
  UnitConverter : DataTypeConversion  OutDataTypeStr=uint8
  convert_in : FVT_lib/hal/convert_in  gain=0.1  offset=0
  VHAL_FrMCUBATNidec_V : Outport
  wires:
  convert_in/1 -> VHAL_FrMCUBATNidec_V/1
  UnitConverter/1 -> convert_in/1
  Fr_MCUBAT_Nidec/1 -> UnitConverter/1

== system halin/HAL_IN/CAN3/MCU_N_F1/FrMCUDCBusCurrNidec ==
  Fr_MCUDCBusCurr_Nidec : Inport
  UnitConverter : DataTypeConversion  OutDataTypeStr=uint16
  convert_in : FVT_lib/hal/convert_in  gain=0.1  offset=-1500
  VHAL_FrMCUDCBusCurrNidec_A : Outport
  wires:
  convert_in/1 -> VHAL_FrMCUDCBusCurrNidec_A/1
  UnitConverter/1 -> convert_in/1
  Fr_MCUDCBusCurr_Nidec/1 -> UnitConverter/1

== system halin/HAL_IN/CAN3/MCU_N_F1/FrMCUDCBusVoltNidec ==
  Fr_MCUDCBusVolt_Nidec : Inport
  UnitConverter : DataTypeConversion  OutDataTypeStr=uint16
  convert_in : FVT_lib/hal/convert_in  gain=0.1  offset=0
  VHAL_FrMCUDCBusVoltNidec_V : Outport
  wires:
  convert_in/1 -> VHAL_FrMCUDCBusVoltNidec_V/1
  UnitConverter/1 -> convert_in/1
  Fr_MCUDCBusVolt_Nidec/1 -> UnitConverter/1

== system halin/HAL_IN/CAN3/MCU_N_F1/FrMCUDischrgStaNidec ==
  Fr_MCUDischrgSta_Nidec : Inport
  UnitConverter : DataTypeConversion  OutDataTypeStr=uint8
  VHAL_FrMCUDischrgStaNidec_flg : Outport
  wires:
  UnitConverter/1 -> VHAL_FrMCUDischrgStaNidec_flg/1
  Fr_MCUDischrgSta_Nidec/1 -> UnitConverter/1

== system halin/HAL_IN/CAN3/MCU_N_F1/FrMCUEnaStaNidec ==
  Fr_MCUEnaSta_Nidec : Inport
  UnitConverter : DataTypeConversion  OutDataTypeStr=uint8
  VHAL_FrMCUEnaStaNidec_flg : Outport
  wires:
  UnitConverter/1 -> VHAL_FrMCUEnaStaNidec_flg/1
  Fr_MCUEnaSta_Nidec/1 -> UnitConverter/1

== system halin/HAL_IN/CAN3/MCU_N_F1/FrMCUErrNidec ==
  Fr_MCUErr_Nidec : Inport
  UnitConverter : DataTypeConversion  OutDataTypeStr=uint8
  VHAL_FrMCUErrNidec_enum : Outport
  wires:
  UnitConverter/1 -> VHAL_FrMCUErrNidec_enum/1
  Fr_MCUErr_Nidec/1 -> UnitConverter/1

== system halin/HAL_IN/CAN3/MCU_N_F1/FrMCUIGNstaNidec ==
  Fr_MCUIGN_sta_Nidec : Inport
  UnitConverter : DataTypeConversion  OutDataTypeStr=uint8
  VHAL_FrMCUIGNstaNidec_flg : Outport
  wires:
  UnitConverter/1 -> VHAL_FrMCUIGNstaNidec_flg/1
  Fr_MCUIGN_sta_Nidec/1 -> UnitConverter/1

== system halin/HAL_IN/CAN3/MCU_N_F1/FrMCUReady4PreNidec ==
  Fr_MCUReady4Pre_Nidec : Inport
  UnitConverter : DataTypeConversion  OutDataTypeStr=uint8
  VHAL_FrMCUReady4PreNidec_flg : Outport
  wires:
  UnitConverter/1 -> VHAL_FrMCUReady4PreNidec_flg/1
  Fr_MCUReady4Pre_Nidec/1 -> UnitConverter/1

== system halin/HAL_IN/CAN3/MCU_N_F1/FrMCUReadyNidec ==
  Fr_MCUReady_Nidec : Inport
  UnitConverter : DataTypeConversion  OutDataTypeStr=uint8
  VHAL_FrMCUReadyNidec_flg : Outport
  wires:
  UnitConverter/1 -> VHAL_FrMCUReadyNidec_flg/1
  Fr_MCUReady_Nidec/1 -> UnitConverter/1

== system halin/HAL_IN/CAN3/MCU_N_F1/FrMCUSysStaNidec ==
  Fr_MCUSysSta_Nidec : Inport
  UnitConverter : DataTypeConversion  OutDataTypeStr=uint8
  VHAL_FrMCUSysStaNidec_enum : Outport
  wires:
  UnitConverter/1 -> VHAL_FrMCUSysStaNidec_enum/1
  Fr_MCUSysSta_Nidec/1 -> UnitConverter/1

== system halin/HAL_IN/CAN3/MCU_N_F1/FrMCUTempNidec ==
  Fr_MCUTemp_Nidec : Inport
  UnitConverter : DataTypeConversion  OutDataTypeStr=uint16
  convert_in : FVT_lib/hal/convert_in  gain=1  offset=-40
  VHAL_FrMCUTempNidec_C : Outport
  wires:
  convert_in/1 -> VHAL_FrMCUTempNidec_C/1
  UnitConverter/1 -> convert_in/1
  Fr_MCUTemp_Nidec/1 -> UnitConverter/1

== system halin/HAL_IN/CAN3/MCU_N_F1/FrMotorAvailTqNidec ==
  Fr_MotorAvailTq_Nidec : Inport
  UnitConverter : DataTypeConversion  OutDataTypeStr=uint16
  VHAL_FrMotorAvailTqNidec_Nm : Outport
  wires:
  UnitConverter/1 -> VHAL_FrMotorAvailTqNidec_Nm/1
  Fr_MotorAvailTq_Nidec/1 -> UnitConverter/1

== system halin/HAL_IN/CAN3/MCU_N_F1/FrRegenAvailTqNidec ==
  Fr_RegenAvailTq_Nidec : Inport
  UnitConverter : DataTypeConversion  OutDataTypeStr=uint16
  convert_in : FVT_lib/hal/convert_in  gain=1  offset=-1022
  VHAL_FrRegenAvailTqNidec_Nm : Outport
  wires:
  convert_in/1 -> VHAL_FrRegenAvailTqNidec_Nm/1
  UnitConverter/1 -> convert_in/1
  Fr_RegenAvailTq_Nidec/1 -> UnitConverter/1

== system halin/HAL_IN/CAN3/MCU_N_F1/FrTMSpdNidec ==
  Fr_TMSpd_Nidec : Inport
  UnitConverter : DataTypeConversion  OutDataTypeStr=uint16
  convert_in : FVT_lib/hal/convert_in  gain=1  offset=-17000
  VHAL_FrTMSpdNidec_rpm : Outport
  wires:
  convert_in/1 -> VHAL_FrTMSpdNidec_rpm/1
  UnitConverter/1 -> convert_in/1
  Fr_TMSpd_Nidec/1 -> UnitConverter/1

== system halin/HAL_IN/CAN3/MCU_N_F1/FrTMTempNidec ==
  Fr_TMTemp_Nidec : Inport
  UnitConverter : DataTypeConversion  OutDataTypeStr=uint16
  convert_in : FVT_lib/hal/convert_in  gain=1  offset=-40
  VHAL_FrTMTempNidec_C : Outport
  wires:
  convert_in/1 -> VHAL_FrTMTempNidec_C/1
  UnitConverter/1 -> convert_in/1
  Fr_TMTemp_Nidec/1 -> UnitConverter/1

== system halin/HAL_IN/CAN3/MCU_N_F1/FrTMidNidec ==
  Fr_TMid_Nidec : Inport
  UnitConverter : DataTypeConversion  OutDataTypeStr=uint16
  convert_in : FVT_lib/hal/convert_in  gain=0.1  offset=-1500
  VHAL_FrTMidNidec_A : Outport
  wires:
  convert_in/1 -> VHAL_FrTMidNidec_A/1
  UnitConverter/1 -> convert_in/1
  Fr_TMid_Nidec/1 -> UnitConverter/1

== system halin/HAL_IN/CAN3/MCU_N_F1/FrTMiqNidec ==
  Fr_TMiq_Nidec : Inport
  UnitConverter : DataTypeConversion  OutDataTypeStr=uint16
  convert_in : FVT_lib/hal/convert_in  gain=0.1  offset=-1500
  VHAL_FrTMiqNidec_A : Outport
  wires:
  convert_in/1 -> VHAL_FrTMiqNidec_A/1
  UnitConverter/1 -> convert_in/1
  Fr_TMiq_Nidec/1 -> UnitConverter/1

== system halin/HAL_IN/CAN3/MCU_N_F1/MCUWarnFNidec ==
  MCUWarn_F_Nidec : Inport
  UnitConverter : DataTypeConversion  OutDataTypeStr=uint8
  VHAL_MCUWarnFNidec_enum : Outport
  wires:
  UnitConverter/1 -> VHAL_MCUWarnFNidec_enum/1
  MCUWarn_F_Nidec/1 -> UnitConverter/1

== system halin/HAL_IN/CAN3/MCU_N_F2/FrCoolanttempReqNidec ==
  Fr_CoolanttempReq_Nidec : Inport
  UnitConverter : DataTypeConversion  OutDataTypeStr=uint16
  convert_in : FVT_lib/hal/convert_in  gain=1  offset=-40
  VHAL_FrCoolanttempReqNidec_C : Outport
  wires:
  convert_in/1 -> VHAL_FrCoolanttempReqNidec_C/1
  UnitConverter/1 -> convert_in/1
  Fr_CoolanttempReq_Nidec/1 -> UnitConverter/1

== system halin/HAL_IN/CAN3/MCU_N_F2/FrEOPSpdSetNidec ==
  Fr_EOP_SpdSet_Nidec : Inport
  UnitConverter : DataTypeConversion  OutDataTypeStr=uint16
  VHAL_FrEOPSpdSetNidec_rpm : Outport
  wires:
  UnitConverter/1 -> VHAL_FrEOPSpdSetNidec_rpm/1
  Fr_EOP_SpdSet_Nidec/1 -> UnitConverter/1

== system halin/HAL_IN/CAN3/MCU_N_F2/FrFailcode1Nidec ==
  Fr_Failcode1_Nidec : Inport
  UnitConverter : DataTypeConversion  OutDataTypeStr=uint8
  VHAL_FrFailcode1Nidec_enum : Outport
  wires:
  UnitConverter/1 -> VHAL_FrFailcode1Nidec_enum/1
  Fr_Failcode1_Nidec/1 -> UnitConverter/1

== system halin/HAL_IN/CAN3/MCU_N_F2/FrFailcode2Nidec ==
  Fr_Failcode2_Nidec : Inport
  UnitConverter : DataTypeConversion  OutDataTypeStr=uint8
  VHAL_FrFailcode2Nidec_enum : Outport
  wires:
  UnitConverter/1 -> VHAL_FrFailcode2Nidec_enum/1
  Fr_Failcode2_Nidec/1 -> UnitConverter/1

== system halin/HAL_IN/CAN3/MCU_N_F2/FrFailcodehistory1Nidec ==
  Fr_Failcodehistory1_Nidec : Inport
  UnitConverter : DataTypeConversion  OutDataTypeStr=uint8
  VHAL_FrFailcodehistory1Nidec_enum : Outport
  wires:
  UnitConverter/1 -> VHAL_FrFailcodehistory1Nidec_enum/1
  Fr_Failcodehistory1_Nidec/1 -> UnitConverter/1

== system halin/HAL_IN/CAN3/MCU_N_F2/FrFailcodehistory2Nidec ==
  Fr_Failcodehistory2_Nidec : Inport
  UnitConverter : DataTypeConversion  OutDataTypeStr=uint8
  VHAL_FrFailcodehistory2Nidec_enum : Outport
  wires:
  UnitConverter/1 -> VHAL_FrFailcodehistory2Nidec_enum/1
  Fr_Failcodehistory2_Nidec/1 -> UnitConverter/1

== system halin/HAL_IN/CAN3/MCU_N_F2/FrLLCTempNidec ==
  Fr_LLCTemp_Nidec : Inport
  UnitConverter : DataTypeConversion  OutDataTypeStr=uint16
  convert_in : FVT_lib/hal/convert_in  gain=1  offset=-40
  VHAL_FrLLCTempNidec_C : Outport
  wires:
  convert_in/1 -> VHAL_FrLLCTempNidec_C/1
  UnitConverter/1 -> convert_in/1
  Fr_LLCTemp_Nidec/1 -> UnitConverter/1

== system halin/HAL_IN/CAN3/MCU_N_F2/FrLLCflowReqNidec ==
  Fr_LLCflowReq_Nidec : Inport
  UnitConverter : DataTypeConversion  OutDataTypeStr=uint8
  convert_in : FVT_lib/hal/convert_in  gain=0.25  offset=0
  VHAL_FrLLCflowReqNidec_Lpmin : Outport
  wires:
  convert_in/1 -> VHAL_FrLLCflowReqNidec_Lpmin/1
  UnitConverter/1 -> convert_in/1
  Fr_LLCflowReq_Nidec/1 -> UnitConverter/1

== system halin/HAL_IN/CAN3/MCU_N_F2/FrMCUTempWarnNidec ==
  Fr_MCUTempWarn_Nidec : Inport
  UnitConverter : DataTypeConversion  OutDataTypeStr=uint8
  VHAL_FrMCUTempWarnNidec_enum : Outport
  wires:
  UnitConverter/1 -> VHAL_FrMCUTempWarnNidec_enum/1
  Fr_MCUTempWarn_Nidec/1 -> UnitConverter/1

== system halin/HAL_IN/CAN3/MCU_N_F2/FrTMTempWarnNidec ==
  Fr_TMTempWarn_Nidec : Inport
  UnitConverter : DataTypeConversion  OutDataTypeStr=uint8
  VHAL_FrTMTempWarnNidec_enum : Outport
  wires:
  UnitConverter/1 -> VHAL_FrTMTempWarnNidec_enum/1
  Fr_TMTempWarn_Nidec/1 -> UnitConverter/1

== system halin/HAL_IN/CAN3/MCU_N_F3/FrMCUHWVerNidec ==
  Fr_MCU_HW_Ver_Nidec : Inport
  UnitConverter : DataTypeConversion  OutDataTypeStr=uint16
  VHAL_FrMCUHWVerNidec_enum : Outport
  wires:
  UnitConverter/1 -> VHAL_FrMCUHWVerNidec_enum/1
  Fr_MCU_HW_Ver_Nidec/1 -> UnitConverter/1

== system halin/HAL_IN/CAN3/MCU_N_F3/FrMCUSWVerNidec ==
  Fr_MCU_SW_Ver_Nidec : Inport
  UnitConverter : DataTypeConversion  OutDataTypeStr=uint16
  VHAL_FrMCUSWVerNidec_enum : Outport
  wires:
  UnitConverter/1 -> VHAL_FrMCUSWVerNidec_enum/1
  Fr_MCU_SW_Ver_Nidec/1 -> UnitConverter/1

== system halin/HAL_IN/CAN3/MCU_N_R1/MCUWarnRNidec ==
  MCUWarn_R_Nidec : Inport
  UnitConverter : DataTypeConversion  OutDataTypeStr=uint8
  VHAL_MCUWarnRNidec_enum : Outport
  wires:
  UnitConverter/1 -> VHAL_MCUWarnRNidec_enum/1
  MCUWarn_R_Nidec/1 -> UnitConverter/1

== system halin/HAL_IN/CAN3/MCU_N_R1/RrActvDmpDisabStaNidec ==
  Rr_ActvDmpDisabSta_Nidec : Inport
  UnitConverter : DataTypeConversion  OutDataTypeStr=uint8
  VHAL_RrActvDmpDisabStaNidec_flg : Outport
  wires:
  UnitConverter/1 -> VHAL_RrActvDmpDisabStaNidec_flg/1
  Rr_ActvDmpDisabSta_Nidec/1 -> UnitConverter/1

== system halin/HAL_IN/CAN3/MCU_N_R1/RrEDUDrtStaNidec ==
  Rr_EDUDrtSta_Nidec : Inport
  UnitConverter : DataTypeConversion  OutDataTypeStr=uint8
  VHAL_RrEDUDrtStaNidec_flg : Outport
  wires:
  UnitConverter/1 -> VHAL_RrEDUDrtStaNidec_flg/1
  Rr_EDUDrtSta_Nidec/1 -> UnitConverter/1

== system halin/HAL_IN/CAN3/MCU_N_R1/RrEDUOpratingStaNidec ==
  Rr_EDUOpratingSta_Nidec : Inport
  UnitConverter : DataTypeConversion  OutDataTypeStr=uint8
  VHAL_RrEDUOpratingStaNidec_flg : Outport
  wires:
  UnitConverter/1 -> VHAL_RrEDUOpratingStaNidec_flg/1
  Rr_EDUOpratingSta_Nidec/1 -> UnitConverter/1

== system halin/HAL_IN/CAN3/MCU_N_R1/RrEDURealTMTqNidec ==
  Rr_EDURealTMTq_Nidec : Inport
  UnitConverter : DataTypeConversion  OutDataTypeStr=uint16
  convert_in : FVT_lib/hal/convert_in  gain=1  offset=-1022
  VHAL_RrEDURealTMTqNidec_Nm : Outport
  wires:
  convert_in/1 -> VHAL_RrEDURealTMTqNidec_Nm/1
  UnitConverter/1 -> convert_in/1
  Rr_EDURealTMTq_Nidec/1 -> UnitConverter/1

== system halin/HAL_IN/CAN3/MCU_N_R1/RrEDURotateDirctionNidec ==
  Rr_EDURotateDirction_Nidec : Inport
  UnitConverter : DataTypeConversion  OutDataTypeStr=uint8
  VHAL_RrEDURotateDirctionNidec_enum : Outport
  wires:
  UnitConverter/1 -> VHAL_RrEDURotateDirctionNidec_enum/1
  Rr_EDURotateDirction_Nidec/1 -> UnitConverter/1

== system halin/HAL_IN/CAN3/MCU_N_R1/RrEDUTqReqFbkNidec ==
  Rr_EDUTqReqFbk_Nidec : Inport
  UnitConverter : DataTypeConversion  OutDataTypeStr=uint16
  convert_in : FVT_lib/hal/convert_in  gain=1  offset=-1022
  VHAL_RrEDUTqReqFbkNidec_Nm : Outport
  wires:
  convert_in/1 -> VHAL_RrEDUTqReqFbkNidec_Nm/1
  UnitConverter/1 -> convert_in/1
  Rr_EDUTqReqFbk_Nidec/1 -> UnitConverter/1

== system halin/HAL_IN/CAN3/MCU_N_R1/RrMCU1ChksumNidec ==
  Rr_MCU1Chksum_Nidec : Inport
  UnitConverter : DataTypeConversion  OutDataTypeStr=uint8
  VHAL_RrMCU1ChksumNidec_enum : Outport
  wires:
  UnitConverter/1 -> VHAL_RrMCU1ChksumNidec_enum/1
  Rr_MCU1Chksum_Nidec/1 -> UnitConverter/1

== system halin/HAL_IN/CAN3/MCU_N_R1/RrMCU1RolCntNidec ==
  Rr_MCU1RolCnt_Nidec : Inport
  UnitConverter : DataTypeConversion  OutDataTypeStr=uint8
  VHAL_RrMCU1RolCntNidec_enum : Outport
  wires:
  UnitConverter/1 -> VHAL_RrMCU1RolCntNidec_enum/1
  Rr_MCU1RolCnt_Nidec/1 -> UnitConverter/1

== system halin/HAL_IN/CAN3/MCU_N_R1/RrMCUBATNidec ==
  Rr_MCUBAT_Nidec : Inport
  UnitConverter : DataTypeConversion  OutDataTypeStr=uint8
  convert_in : FVT_lib/hal/convert_in  gain=0.1  offset=0
  VHAL_RrMCUBATNidec_V : Outport
  wires:
  convert_in/1 -> VHAL_RrMCUBATNidec_V/1
  UnitConverter/1 -> convert_in/1
  Rr_MCUBAT_Nidec/1 -> UnitConverter/1

== system halin/HAL_IN/CAN3/MCU_N_R1/RrMCUDCBusCurrNidec ==
  Rr_MCUDCBusCurr_Nidec : Inport
  UnitConverter : DataTypeConversion  OutDataTypeStr=uint16
  convert_in : FVT_lib/hal/convert_in  gain=0.1  offset=-1500
  VHAL_RrMCUDCBusCurrNidec_A : Outport
  wires:
  convert_in/1 -> VHAL_RrMCUDCBusCurrNidec_A/1
  UnitConverter/1 -> convert_in/1
  Rr_MCUDCBusCurr_Nidec/1 -> UnitConverter/1

== system halin/HAL_IN/CAN3/MCU_N_R1/RrMCUDCBusVoltNidec ==
  Rr_MCUDCBusVolt_Nidec : Inport
  UnitConverter : DataTypeConversion  OutDataTypeStr=uint16
  convert_in : FVT_lib/hal/convert_in  gain=0.1  offset=0
  VHAL_RrMCUDCBusVoltNidec_V : Outport
  wires:
  convert_in/1 -> VHAL_RrMCUDCBusVoltNidec_V/1
  UnitConverter/1 -> convert_in/1
  Rr_MCUDCBusVolt_Nidec/1 -> UnitConverter/1

== system halin/HAL_IN/CAN3/MCU_N_R1/RrMCUDischrgStaNidec ==
  Rr_MCUDischrgSta_Nidec : Inport
  UnitConverter : DataTypeConversion  OutDataTypeStr=uint8
  VHAL_RrMCUDischrgStaNidec_flg : Outport
  wires:
  UnitConverter/1 -> VHAL_RrMCUDischrgStaNidec_flg/1
  Rr_MCUDischrgSta_Nidec/1 -> UnitConverter/1

== system halin/HAL_IN/CAN3/MCU_N_R1/RrMCUEnaStaNidec ==
  Rr_MCUEnaSta_Nidec : Inport
  UnitConverter : DataTypeConversion  OutDataTypeStr=uint8
  VHAL_RrMCUEnaStaNidec_flg : Outport
  wires:
  UnitConverter/1 -> VHAL_RrMCUEnaStaNidec_flg/1
  Rr_MCUEnaSta_Nidec/1 -> UnitConverter/1

== system halin/HAL_IN/CAN3/MCU_N_R1/RrMCUErrNidec ==
  Rr_MCUErr_Nidec : Inport
  UnitConverter : DataTypeConversion  OutDataTypeStr=uint8
  VHAL_RrMCUErrNidec_enum : Outport
  wires:
  UnitConverter/1 -> VHAL_RrMCUErrNidec_enum/1
  Rr_MCUErr_Nidec/1 -> UnitConverter/1

== system halin/HAL_IN/CAN3/MCU_N_R1/RrMCUIGNstaNidec ==
  Rr_MCUIGN_sta_Nidec : Inport
  UnitConverter : DataTypeConversion  OutDataTypeStr=uint8
  VHAL_RrMCUIGNstaNidec_flg : Outport
  wires:
  UnitConverter/1 -> VHAL_RrMCUIGNstaNidec_flg/1
  Rr_MCUIGN_sta_Nidec/1 -> UnitConverter/1

== system halin/HAL_IN/CAN3/MCU_N_R1/RrMCUReady4PreNidec ==
  Rr_MCUReady4Pre_Nidec : Inport
  UnitConverter : DataTypeConversion  OutDataTypeStr=uint8
  VHAL_RrMCUReady4PreNidec_flg : Outport
  wires:
  UnitConverter/1 -> VHAL_RrMCUReady4PreNidec_flg/1
  Rr_MCUReady4Pre_Nidec/1 -> UnitConverter/1

== system halin/HAL_IN/CAN3/MCU_N_R1/RrMCUReadyNidec ==
  Rr_MCUReady_Nidec : Inport
  UnitConverter : DataTypeConversion  OutDataTypeStr=uint8
  VHAL_RrMCUReadyNidec_flg : Outport
  wires:
  UnitConverter/1 -> VHAL_RrMCUReadyNidec_flg/1
  Rr_MCUReady_Nidec/1 -> UnitConverter/1

== system halin/HAL_IN/CAN3/MCU_N_R1/RrMCUSysStaNidec ==
  Rr_MCUSysSta_Nidec : Inport
  UnitConverter : DataTypeConversion  OutDataTypeStr=uint8
  VHAL_RrMCUSysStaNidec_enum : Outport
  wires:
  UnitConverter/1 -> VHAL_RrMCUSysStaNidec_enum/1
  Rr_MCUSysSta_Nidec/1 -> UnitConverter/1

== system halin/HAL_IN/CAN3/MCU_N_R1/RrMCUTempNidec ==
  Rr_MCUTemp_Nidec : Inport
  UnitConverter : DataTypeConversion  OutDataTypeStr=uint16
  convert_in : FVT_lib/hal/convert_in  gain=1  offset=-40
  VHAL_RrMCUTempNidec_C : Outport
  wires:
  convert_in/1 -> VHAL_RrMCUTempNidec_C/1
  UnitConverter/1 -> convert_in/1
  Rr_MCUTemp_Nidec/1 -> UnitConverter/1

== system halin/HAL_IN/CAN3/MCU_N_R1/RrMotorAvailTqNidec ==
  Rr_MotorAvailTq_Nidec : Inport
  UnitConverter : DataTypeConversion  OutDataTypeStr=uint16
  VHAL_RrMotorAvailTqNidec_Nm : Outport
  wires:
  UnitConverter/1 -> VHAL_RrMotorAvailTqNidec_Nm/1
  Rr_MotorAvailTq_Nidec/1 -> UnitConverter/1

== system halin/HAL_IN/CAN3/MCU_N_R1/RrRegenAvailTqNidec ==
  Rr_RegenAvailTq_Nidec : Inport
  UnitConverter : DataTypeConversion  OutDataTypeStr=uint16
  convert_in : FVT_lib/hal/convert_in  gain=1  offset=-1022
  VHAL_RrRegenAvailTqNidec_Nm : Outport
  wires:
  convert_in/1 -> VHAL_RrRegenAvailTqNidec_Nm/1
  UnitConverter/1 -> convert_in/1
  Rr_RegenAvailTq_Nidec/1 -> UnitConverter/1

== system halin/HAL_IN/CAN3/MCU_N_R1/RrTMSpdNidec ==
  Rr_TMSpd_Nidec : Inport
  UnitConverter : DataTypeConversion  OutDataTypeStr=uint16
  convert_in : FVT_lib/hal/convert_in  gain=1  offset=-17000
  VHAL_RrTMSpdNidec_rpm : Outport
  wires:
  convert_in/1 -> VHAL_RrTMSpdNidec_rpm/1
  UnitConverter/1 -> convert_in/1
  Rr_TMSpd_Nidec/1 -> UnitConverter/1

== system halin/HAL_IN/CAN3/MCU_N_R1/RrTMTempNidec ==
  Rr_TMTemp_Nidec : Inport
  UnitConverter : DataTypeConversion  OutDataTypeStr=uint16
  convert_in : FVT_lib/hal/convert_in  gain=1  offset=-40
  VHAL_RrTMTempNidec_C : Outport
  wires:
  convert_in/1 -> VHAL_RrTMTempNidec_C/1
  UnitConverter/1 -> convert_in/1
  Rr_TMTemp_Nidec/1 -> UnitConverter/1

== system halin/HAL_IN/CAN3/MCU_N_R1/RrTMidNidec ==
  Rr_TMid_Nidec : Inport
  UnitConverter : DataTypeConversion  OutDataTypeStr=uint16
  convert_in : FVT_lib/hal/convert_in  gain=0.1  offset=-1500
  VHAL_RrTMidNidec_A : Outport
  wires:
  convert_in/1 -> VHAL_RrTMidNidec_A/1
  UnitConverter/1 -> convert_in/1
  Rr_TMid_Nidec/1 -> UnitConverter/1

== system halin/HAL_IN/CAN3/MCU_N_R1/RrTMiqNidec ==
  Rr_TMiq_Nidec : Inport
  UnitConverter : DataTypeConversion  OutDataTypeStr=uint16
  convert_in : FVT_lib/hal/convert_in  gain=0.1  offset=-1500
  VHAL_RrTMiqNidec_A : Outport
  wires:
  convert_in/1 -> VHAL_RrTMiqNidec_A/1
  UnitConverter/1 -> convert_in/1
  Rr_TMiq_Nidec/1 -> UnitConverter/1

== system halin/HAL_IN/CAN3/MCU_N_R2/RrCoolanttempReqNidec ==
  Rr_CoolanttempReq_Nidec : Inport
  UnitConverter : DataTypeConversion  OutDataTypeStr=uint16
  convert_in : FVT_lib/hal/convert_in  gain=1  offset=-40
  VHAL_RrCoolanttempReqNidec_cnt : Outport
  wires:
  convert_in/1 -> VHAL_RrCoolanttempReqNidec_cnt/1
  UnitConverter/1 -> convert_in/1
  Rr_CoolanttempReq_Nidec/1 -> UnitConverter/1

== system halin/HAL_IN/CAN3/MCU_N_R2/RrEOPSpdSetNidec ==
  Rr_EOP_SpdSet_Nidec : Inport
  UnitConverter : DataTypeConversion  OutDataTypeStr=uint16
  VHAL_RrEOPSpdSetNidec_rpm : Outport
  wires:
  UnitConverter/1 -> VHAL_RrEOPSpdSetNidec_rpm/1
  Rr_EOP_SpdSet_Nidec/1 -> UnitConverter/1

== system halin/HAL_IN/CAN3/MCU_N_R2/RrFailcode1Nidec ==
  Rr_Failcode1_Nidec : Inport
  UnitConverter : DataTypeConversion  OutDataTypeStr=uint8
  VHAL_RrFailcode1Nidec_enum : Outport
  wires:
  UnitConverter/1 -> VHAL_RrFailcode1Nidec_enum/1
  Rr_Failcode1_Nidec/1 -> UnitConverter/1

== system halin/HAL_IN/CAN3/MCU_N_R2/RrFailcode2Nidec ==
  Rr_Failcode2_Nidec : Inport
  UnitConverter : DataTypeConversion  OutDataTypeStr=uint8
  VHAL_RrFailcode2Nidec_enum : Outport
  wires:
  UnitConverter/1 -> VHAL_RrFailcode2Nidec_enum/1
  Rr_Failcode2_Nidec/1 -> UnitConverter/1

== system halin/HAL_IN/CAN3/MCU_N_R2/RrFailcodehistory1Nidec ==
  Rr_Failcodehistory1_Nidec : Inport
  UnitConverter : DataTypeConversion  OutDataTypeStr=uint8
  VHAL_RrFailcodehistory1Nidec_enum : Outport
  wires:
  UnitConverter/1 -> VHAL_RrFailcodehistory1Nidec_enum/1
  Rr_Failcodehistory1_Nidec/1 -> UnitConverter/1

== system halin/HAL_IN/CAN3/MCU_N_R2/RrFailcodehistory2Nidec ==
  Rr_Failcodehistory2_Nidec : Inport
  UnitConverter : DataTypeConversion  OutDataTypeStr=uint8
  VHAL_RrFailcodehistory2Nidec_enum : Outport
  wires:
  UnitConverter/1 -> VHAL_RrFailcodehistory2Nidec_enum/1
  Rr_Failcodehistory2_Nidec/1 -> UnitConverter/1

== system halin/HAL_IN/CAN3/MCU_N_R2/RrLLCTempNidec ==
  Rr_LLCTemp_Nidec : Inport
  UnitConverter : DataTypeConversion  OutDataTypeStr=uint16
  convert_in : FVT_lib/hal/convert_in  gain=1  offset=-40
  VHAL_RrLLCTempNidec_C : Outport
  wires:
  convert_in/1 -> VHAL_RrLLCTempNidec_C/1
  UnitConverter/1 -> convert_in/1
  Rr_LLCTemp_Nidec/1 -> UnitConverter/1
